simulink model "flightController"  (R2022a)
settings: Solver=ode3  StartTime=0  StopTime=TFinal  FixedStep=Ts  RelTol=1e-3  EnableMultiTasking=on
undefined symbols (not defined in the file): Controller, DiscIntNeverNeededParam, Ts, Vehicle
libraries: vrlib x2, dspfdesign x1
(part 2 of 2)

== system flightController/Flight Controller1/LADRC - Roll ==
  y : Inport
  r : Inport  Port=2
  Demux : Demux  Outputs=3
  Digital Clock : DigitalClock  SampleTime=Ts
  Discrete-Time Integrator : DiscreteIntegrator  InitialCondition=[0 0 0]'  SampleTime=Ts  OutDataTypeStr=single  ICPrevOutput=DiscIntNeverNeededParam  ICPrevScaledInput=DiscIntNeverNeededParam
  Divide : Product  Inputs=*/  OutDataTypeStr=single
  Gain1 : Gain  Gain=2  OutDataTypeStr=single
  GreaterThan : RelationalOperator  Operator=>  OutDataTypeStr=boolean  RndMeth=Simplest  InputSameDT=off
  LESO : MATLAB Function  TreatAsAtomicUnit=on
  Product : Product  OutDataTypeStr=single
  Product1 : Product  OutDataTypeStr=single
  SaturationThrust : Saturate  UpperLimit=4*Controller.totalThrustMaxRelative*Controller.motorsThrustPerMotorMax  LowerLimit=-4*Controller.totalThrustMaxRelative*Controller.motorsThrustPerMotorMax  OutDataTypeStr=single
  Square : Math  Operator=square
  Sum1 : Sum  Inputs=+-|
  Sum2 : Sum  Inputs=|+-
  Sum3 : Sum  Inputs=+-|
  Switch : Switch  Criteria=u2 ~= 0  Threshold=0.1  SaturateOnIntegerOverflow=off  InputSameDT=off
  b : Constant  Value=10000  OutDataTypeStr=single
  t_warm : Constant  Value=0.1  OutDataTypeStr=single
  u_ini : Constant  Value=0  OutDataTypeStr=single
  wc : Constant  Value=12  OutDataTypeStr=single
  wo : Constant  Value=40  OutDataTypeStr=single
  u : Outport
  wires:
  LESO/1(z_dot) -> Discrete-Time Integrator/1
  Discrete-Time Integrator/1 -> LESO/1(z), Demux/1
  Demux/1 -> Sum3/2  "z1"
  Product/1 -> Sum1/1
  Sum1/1 -> Sum2/1  "u_0"
  Demux/3 -> Sum2/2  "z3"
  Sum2/1 -> Divide/1
  Square/1 -> Product/1
  Gain1/1 -> Product1/1
  Demux/2 -> Product1/2  "z2"
  Product1/1 -> Sum1/2
  SaturationThrust/1 -> LESO/5(u), u/1  "u"
  Switch/1 -> SaturationThrust/1
  Divide/1 -> Switch/1  "u"
  u_ini/1 -> Switch/3
  r/1 -> Sum3/1
  Sum3/1 -> Product/2
  b/1 -> LESO/3(b), Divide/2
  wc/1 -> Gain1/1, Square/1
  wo/1 -> LESO/2(wo)
  t_warm/1 -> GreaterThan/2
  Digital Clock/1 -> GreaterThan/1
  GreaterThan/1 -> Switch/2
  y/1 -> LESO/4(y)

== system flightController/Flight Controller1/LADRC - Yaw ==
  y : Inport
  r : Inport  Port=2
  Demux : Demux  Outputs=3
  Digital Clock : DigitalClock  SampleTime=Ts
  Discrete-Time Integrator : DiscreteIntegrator  InitialCondition=[0 0 0]'  SampleTime=Ts  OutDataTypeStr=single  ICPrevOutput=DiscIntNeverNeededParam  ICPrevScaledInput=DiscIntNeverNeededParam
  Divide : Product  Inputs=*/  OutDataTypeStr=single
  Gain1 : Gain  Gain=2  OutDataTypeStr=single
  GreaterThan : RelationalOperator  Operator=>  OutDataTypeStr=boolean  RndMeth=Simplest  InputSameDT=off
  LESO : MATLAB Function  TreatAsAtomicUnit=on
  Product : Product  OutDataTypeStr=single
  Product1 : Product  OutDataTypeStr=single
  SaturationThrust : Saturate  Commented=through  UpperLimit=0.001  LowerLimit=-0.001  OutDataTypeStr=single
  Scope : Scope  NumInputPorts=2
  Scope1 : Scope
  Square : Math  Operator=square
  Sum1 : Sum  Inputs=+-|
  Sum2 : Sum  Inputs=|+-
  Sum3 : Sum  Inputs=+-|
  Switch : Switch  Criteria=u2 ~= 0  Threshold=0.1  SaturateOnIntegerOverflow=off  InputSameDT=off
  b : Constant  Value=15000  OutDataTypeStr=single
  t_warm : Constant  Value=0.2  OutDataTypeStr=single
  u_ini : Constant  Value=0  OutDataTypeStr=single
  wc : Constant  Value=4  OutDataTypeStr=single
  wo : Constant  Value=14  OutDataTypeStr=single
  u : Outport
  wires:
  LESO/1(z_dot) -> Discrete-Time Integrator/1
  Discrete-Time Integrator/1 -> LESO/1(z), Demux/1
  Demux/1 -> Scope/1, Sum3/2  "z1"
  Product/1 -> Sum1/1
  Sum1/1 -> Sum2/1  "u_0"
  Demux/3 -> Sum2/2  "z3"
  Sum2/1 -> Divide/1
  Square/1 -> Product/1
  Gain1/1 -> Product1/1
  Demux/2 -> Product1/2  "z2"
  Product1/1 -> Sum1/2
  SaturationThrust/1 -> Scope1/1, LESO/5(u), u/1  "u"
  Switch/1 -> SaturationThrust/1
  Divide/1 -> Switch/1  "u"
  u_ini/1 -> Switch/3
  r/1 -> Sum3/1
  Sum3/1 -> Product/2
  b/1 -> Divide/2, LESO/3(b)
  wc/1 -> Gain1/1, Square/1
  wo/1 -> LESO/2(wo)
  t_warm/1 -> GreaterThan/2
  Digital Clock/1 -> GreaterThan/1
  GreaterThan/1 -> Switch/2
  y/1 -> Scope/2, LESO/4(y)

== system flightController/Flight Controller1/LADRC - dX ==
  y : Inport
  r : Inport  Port=2
  Constant : Constant  OutDataTypeStr=single
  Demux : Demux  Outputs=2
  Digital Clock : DigitalClock  SampleTime=Ts
  Discrete-Time Integrator : DiscreteIntegrator  InitialCondition=[0 0]'  SampleTime=Ts  ICPrevOutput=DiscIntNeverNeededParam  ICPrevScaledInput=DiscIntNeverNeededParam
  Divide : Product  Inputs=*/
  GreaterThan : RelationalOperator  Operator=>  OutDataTypeStr=boolean  RndMeth=Simplest  InputSameDT=off
  LESO - 1st order : MATLAB Function  TreatAsAtomicUnit=on
  Product : Product
  Saturation : Saturate  UpperLimit=pi/8  LowerLimit=-pi/8
  Sum1 : Sum  Inputs=+-|
  Sum3 : Sum  Inputs=+-|
  Switch : Switch  Criteria=u2 ~= 0  Threshold=0.1  SaturateOnIntegerOverflow=off  InputSameDT=off
  b : Gain  Gain=-20
  b1 : Gain  Gain=-30
  bw_c : Gain
  bw_c1 : Gain  Gain=2
  bw_o : Gain  Gain=3
  bw_o1 : Gain  Gain=6
  t_warm : Constant  Value=0.01
  u_ini : Constant  Value=0  OutDataTypeStr=single
  u : Outport
  wires:
  LESO - 1st order/1(z_dot) -> Discrete-Time Integrator/1
  Discrete-Time Integrator/1 -> LESO - 1st order/1(z), Demux/1
  Demux/1 -> Sum3/2  "z1"
  Product/1 -> Sum1/1
  Sum1/1 -> Divide/1  "u_0"
  Demux/2 -> Sum1/2  "z2"
  Saturation/1 -> u/1, LESO - 1st order/5(u)  "u"
  Divide/1 -> Switch/1  "u"
  u_ini/1 -> Switch/3
  r/1 -> Sum3/1
  Sum3/1 -> Product/2
  b/1 -> LESO - 1st order/3(b), Divide/2
  bw_c/1 -> Product/1
  bw_o/1 -> LESO - 1st order/2(wo)
  t_warm/1 -> GreaterThan/2
  Digital Clock/1 -> GreaterThan/1
  GreaterThan/1 -> Switch/2
  y/1 -> LESO - 1st order/4(y)
  Constant/1 -> bw_o/1, bw_c/1, b/1
  Switch/1 -> Saturation/1  "u"

== system flightController/Flight Controller1/LADRC - dY ==
  y : Inport
  r : Inport  Port=2
  Constant : Constant  OutDataTypeStr=single
  Demux : Demux  Outputs=2
  Digital Clock : DigitalClock  SampleTime=Ts
  Discrete-Time Integrator : DiscreteIntegrator  InitialCondition=[0 0]'  SampleTime=Ts  ICPrevOutput=DiscIntNeverNeededParam  ICPrevScaledInput=DiscIntNeverNeededParam
  Divide : Product  Inputs=*/
  GreaterThan : RelationalOperator  Operator=>  OutDataTypeStr=boolean  RndMeth=Simplest  InputSameDT=off
  LESO - 1st order : MATLAB Function  TreatAsAtomicUnit=on
  Product : Product
  Saturation : Saturate  UpperLimit=pi/8  LowerLimit=-pi/8
  Sum1 : Sum  Inputs=+-|
  Sum3 : Sum  Inputs=+-|
  Switch : Switch  Criteria=u2 ~= 0  Threshold=0.1  SaturateOnIntegerOverflow=off  InputSameDT=off
  b : Gain  Gain=20
  bw_c : Gain
  bw_o : Gain  Gain=3
  t_warm : Constant  Value=0.01
  u_ini : Constant  Value=0  OutDataTypeStr=single
  u : Outport
  wires:
  LESO - 1st order/1(z_dot) -> Discrete-Time Integrator/1
  Discrete-Time Integrator/1 -> LESO - 1st order/1(z), Demux/1
  Demux/1 -> Sum3/2  "z1"
  Product/1 -> Sum1/1
  Sum1/1 -> Divide/1  "u_0"
  Demux/2 -> Sum1/2  "z2"
  Saturation/1 -> u/1, LESO - 1st order/5(u)  "u"
  Divide/1 -> Switch/1  "u"
  u_ini/1 -> Switch/3
  r/1 -> Sum3/1
  Sum3/1 -> Product/2
  b/1 -> LESO - 1st order/3(b), Divide/2
  bw_c/1 -> Product/1
  bw_o/1 -> LESO - 1st order/2(wo)
  t_warm/1 -> GreaterThan/2
  Digital Clock/1 -> GreaterThan/1
  GreaterThan/1 -> Switch/2
  y/1 -> LESO - 1st order/4(y)
  Constant/1 -> bw_o/1, bw_c/1, b/1
  Switch/1 -> Saturation/1  "u"

== system flightController/Flight Controller1/LADRC - dZ ==
  y : Inport
  r : Inport  Port=2
  Demux : Demux  Outputs=3
  Digital Clock : DigitalClock  SampleTime=Ts
  Discrete LESO 2nd Order : MATLAB Function  TreatAsAtomicUnit=on
  Divide : Product  Inputs=*/  OutDataTypeStr=single
  Gain : Gain  Gain=3  OutDataTypeStr=single
  Gain1 : Gain  Gain=2  OutDataTypeStr=single
  GreaterThan : RelationalOperator  Operator=>  OutDataTypeStr=boolean  RndMeth=Simplest  InputSameDT=off
  Magnitude Limit : Saturate  UpperLimit=4*Controller.totalThrustMaxRelative*Controller.motorsThrustPerMotorMax  LowerLimit=-4*Controller.totalThrustMaxRelative*Controller.motorsThrustPerMotorMax  OutDataTypeStr=single
  Memory : Memory  InitialCondition=[0 0 380]'
  Memory1 : Memory  InitialCondition=-0.6
  Product : Product  OutDataTypeStr=single
  Product1 : Product  OutDataTypeStr=single
  Rate Limit : Saturate  UpperLimit=0.05  LowerLimit=-0.05
  Square : Math  Operator=square
  Sum : Sum  Inputs=|++
  Sum1 : Sum  Inputs=+-|
  Sum2 : Sum  Inputs=|+-
  Sum3 : Sum  Inputs=+-|
  Sum4 : Sum  Inputs=|+-
  Switch : Switch  Criteria=u2 ~= 0  Threshold=0.1  SaturateOnIntegerOverflow=off  InputSameDT=off
  b : Constant  Value=800  OutDataTypeStr=single
  t_warm : Constant  Value=0  OutDataTypeStr=single
  u_ini : Constant  Value=-1  OutDataTypeStr=single
  wc : Constant  Value=20  OutDataTypeStr=single
  u : Outport
  wires:
  Discrete LESO 2nd Order/1(z_out) -> Memory/1, Demux/1
  Demux/1 -> Sum3/2  "z1"
  Product/1 -> Sum1/1
  Sum1/1 -> Sum2/1  "u_0"
  Demux/3 -> Sum2/2  "z3"
  Sum2/1 -> Divide/1
  Square/1 -> Product/1
  Gain1/1 -> Product1/1
  Demux/2 -> Product1/2  "z2"
  Product1/1 -> Sum1/2
  Divide/1 -> Switch/1  "u"
  u_ini/1 -> Switch/3
  r/1 -> Sum3/1
  Sum3/1 -> Product/2
  b/1 -> Divide/2, Discrete LESO 2nd Order/2(b)
  wc/1 -> Gain/1, Square/1, Gain1/1
  Gain/1 -> Discrete LESO 2nd Order/3(wo)
  t_warm/1 -> GreaterThan/2
  Digital Clock/1 -> GreaterThan/1
  GreaterThan/1 -> Switch/2
  y/1 -> Discrete LESO 2nd Order/4(y)
  Memory/1 -> Discrete LESO 2nd Order/1(z_in)
  Memory1/1 -> Sum4/2, Discrete LESO 2nd Order/5(u), Sum/2
  Rate Limit/1 -> Sum/1
  Sum/1 -> Magnitude Limit/1
  Sum4/1 -> Rate Limit/1
  Switch/1 -> Sum4/1
  Magnitude Limit/1 -> u/1, Memory1/1

== system flightController/Flight Controller1/LADRC - dZ1 ==
  y : Inport
  r : Inport  Port=2
  Demux : Demux  Outputs=3
  Digital Clock : DigitalClock  SampleTime=Ts
  Discrete LESO 2nd Order : MATLAB Function  TreatAsAtomicUnit=on
  Divide : Product  Inputs=*/  OutDataTypeStr=single
  Gain : Gain  Gain=3  OutDataTypeStr=single
  Gain1 : Gain  Gain=2  OutDataTypeStr=single
  GreaterThan : RelationalOperator  Operator=>  OutDataTypeStr=boolean  RndMeth=Simplest  InputSameDT=off
  Magnitude Limit : Saturate  UpperLimit=4*Controller.totalThrustMaxRelative*Controller.motorsThrustPerMotorMax  LowerLimit=-4*Controller.totalThrustMaxRelative*Controller.motorsThrustPerMotorMax  OutDataTypeStr=single
  Memory : Memory  InitialCondition=[0 0 0]'
  Memory1 : Memory
  Product : Product  OutDataTypeStr=single
  Product1 : Product  OutDataTypeStr=single
  Rate Limit : Saturate  UpperLimit=0.05  LowerLimit=-0.05
  Square : Math  Operator=square
  Sum : Sum  Inputs=|++
  Sum1 : Sum  Inputs=+-|
  Sum2 : Sum  Inputs=|+-
  Sum3 : Sum  Inputs=+-|
  Sum4 : Sum  Inputs=|+-
  Switch : Switch  Criteria=u2 ~= 0  Threshold=0.1  SaturateOnIntegerOverflow=off  InputSameDT=off
  b : Constant  Value=10000  OutDataTypeStr=single
  t_warm : Constant  Value=0  OutDataTypeStr=single
  u_ini : Constant  Value=-1  OutDataTypeStr=single
  wc : Constant  Value=10  OutDataTypeStr=single
  u : Outport
  wires:
  Discrete LESO 2nd Order/1(z_out) -> Memory/1, Demux/1
  Demux/1 -> Sum3/2  "z1"
  Product/1 -> Sum1/1
  Sum1/1 -> Sum2/1  "u_0"
  Demux/3 -> Sum2/2  "z3"
  Sum2/1 -> Divide/1
  Square/1 -> Product/1
  Gain1/1 -> Product1/1
  Demux/2 -> Product1/2  "z2"
  Product1/1 -> Sum1/2
  Divide/1 -> Switch/1  "u"
  u_ini/1 -> Switch/3
  r/1 -> Sum3/1
  Sum3/1 -> Product/2
  b/1 -> Divide/2, Discrete LESO 2nd Order/2(b)
  wc/1 -> Gain/1, Square/1, Gain1/1
  Gain/1 -> Discrete LESO 2nd Order/3(wo)
  t_warm/1 -> GreaterThan/2
  Digital Clock/1 -> GreaterThan/1
  GreaterThan/1 -> Switch/2
  y/1 -> Discrete LESO 2nd Order/4(y)
  Memory/1 -> Discrete LESO 2nd Order/1(z_in)
  Memory1/1 -> Sum4/2, Discrete LESO 2nd Order/5(u), Sum/2
  Rate Limit/1 -> Sum/1
  Sum/1 -> Magnitude Limit/1
  Sum4/1 -> Rate Limit/1
  Switch/1 -> Sum4/1
  Magnitude Limit/1 -> u/1, Memory1/1

== system flightController/Flight Controller1/XBOX CONTROLLER ==
  Bus Creator : BusCreator  Inputs=8
  Bus Creator1 : BusCreator  Inputs=11
  Constant : Constant  Value=[0 0 0 0 0 0 0 0]
  Dead Zone{,1..3} (4 alike) : DeadZone  LowerValue=-0.18  UpperValue=0.18
  Demux : Demux  Outputs=8
  Demux1 : Demux  Outputs=11
  Gain : Gain  Gain=-1
  Gain1 : Gain
  Joystick Input : vrlib/Joystick Input  joyid=1  adjustports=on  forcefeed=off
  Analog : Outport
  Buttons : Outport  Port=2
  wires:
  Demux1/4 -> Bus Creator1/4  "Y"
  Dead Zone/1 -> Bus Creator/1  "LStick-X"
  Demux1/9 -> Bus Creator1/9  "XBOX"
  Demux1/1 -> Bus Creator1/1  "A"
  Demux1/10 -> Bus Creator1/10  "LStick"
  Demux1/5 -> Bus Creator1/5  "LB"
  Demux/7 -> Bus Creator/7  "DPad-X"
  Joystick Input/2 -> Demux1/1
  Demux/5 -> Dead Zone3/1  "RStick-Y"
  Demux/4 -> Dead Zone2/1  "RStick-X"
  Dead Zone2/1 -> Bus Creator/4  "RStick-X"
  Demux/3 -> Bus Creator/3  "LT"
  Demux/8 -> Bus Creator/8  "DPad-Y"
  Joystick Input/1 -> Demux/1
  Demux/6 -> Bus Creator/6  "RT"
  Dead Zone1/1 -> Gain1/1  "LStick-Y"
  Demux/1 -> Dead Zone/1  "LStick-X"
  Bus Creator1/1 -> Buttons/1  "Buttons"
  Gain/1 -> Bus Creator/5  "RStick-Y"
  Demux/2 -> Dead Zone1/1  "LStick-Y"
  Bus Creator/1 -> Analog/1  "Analog"
  Demux1/3 -> Bus Creator1/3  "X"
  Demux1/6 -> Bus Creator1/6  "RB"
  Demux1/7 -> Bus Creator1/7  "Back"
  Demux1/11 -> Bus Creator1/11  "RStick"
  Demux1/2 -> Bus Creator1/2  "B"
  Demux1/8 -> Bus Creator1/8  "Start"
  Dead Zone3/1 -> Gain/1  "RStick-Y"
  Gain1/1 -> Bus Creator/2  "LStick-Y"

== system flightController/Flight Controller1/thrustsToMotorCommands ==
  thrusts_refin : Inport
  1 : Constant  OutDataTypeStr=single
  10 : Constant  Value=10  OutDataTypeStr=single
  2 : Constant  Value=-1  OutDataTypeStr=single
  Digital Clock : DigitalClock  SampleTime=Ts
  Digital Clock1 : DigitalClock  SampleTime=Ts
  Gain : Gain  Gain=1/40  OutDataTypeStr=single
  GreaterThan : RelationalOperator  Operator=>  OutDataTypeStr=boolean  RndMeth=Simplest  InputSameDT=off
  MotorDirections : Gain  Gain=[1 -1 1 -1]
  Mux : Mux
  Product : Product  OutDataTypeStr=single
  Saturation : Saturate  UpperLimit=40  LowerLimit=0  OutDataTypeStr=single
  Saturation5 : Saturate  UpperLimit=Vehicle.Motor.maxLimit  LowerLimit=Vehicle.Motor.minLimit
  Scope : Scope
  Sum : Sum  Inputs=|+-
  Sum1 : Sum  Inputs=|-+
  Switch : Switch  Criteria=u2 ~= 0  Threshold=0.1  SaturateOnIntegerOverflow=off  InputSameDT=off
  ThrustToMotorCommand : Gain  Gain=-Vehicle.Motor.thrustToMotorCommand
  t_warm : Constant  Value=10  OutDataTypeStr=single
  motors_cmdout : Outport  VectorParamsAs1DForOutWhenUnconnected=off
  wires:
  Saturation5/1 -> Product/2, MotorDirections/1
  MotorDirections/1 -> Switch/3
  ThrustToMotorCommand/1 -> Saturation5/1
  thrusts_refin/1 -> ThrustToMotorCommand/1
  Product/1 -> Switch/1
  Switch/1 -> motors_cmdout/1
  GreaterThan/1 -> Switch/2
  Digital Clock/1 -> GreaterThan/1
  t_warm/1 -> GreaterThan/2
  Digital Clock1/1 -> Sum/1
  10/1 -> Sum/2
  Sum/1 -> Saturation/1
  Saturation/1 -> Gain/1
  1/1 -> Mux/3, Sum1/2
  2/1 -> Mux/2, Mux/4
  Sum1/1 -> Scope/1, Mux/1
  Mux/1 -> Product/1

== matlab function flightController/Flight Controller1/LADRC - Roll/LESO ==
  data: z input single size=[3 1]; wo input single; b input single; z_dot output single size=[3 1]; y input single; u input single
function z_dot = LESO(z, wo, b, y, u)
    A = [0 1 0; 0 0 1; 0 0 0];
    B = [0 b 0]';
    C = [1 0 0];
    L = [3*wo 3*wo^2 wo^3]';
        
    z_dot = A*z + B*u + L*(y-z(1));

== matlab function flightController/Flight Controller1/LADRC - Yaw/LESO ==
  data: z input single size=[3 1]; wo input single; b input single; z_dot output single size=[3 1]; y input single; u input single
function z_dot = LESO(z, wo, b, y, u)
    A = [0 1 0; 0 0 1; 0 0 0];
    B = [0 b 0]';
    C = [1 0 0];
    L = [3*wo 3*wo^2 wo^3]';
        
    z_dot = A*z + B*u + L*(y-z(1));

== matlab function flightController/Flight Controller1/LADRC - dX/LESO - 1st order ==
  data: z input single; wo input single; b input single; z_dot output single; y input single; u input single
function z_dot = LESO(z, wo, b, y, u)

% %     A = [zeros(2,1), eye(2); zeros(1,2+1)];
%     A = [0 1 0; 0 0 1; 0 0 0];
% %     B = [zeros(2-1, 1); b; 0];
%     B = [0 1 0]';
% %     L = poly(-wo * ones(1, 2+1));
% %     L = flip(L(2:end));
%     L = []
%     C = [1 0 0];

    A = [0 1; 0 0];
    B = [b 0]';
    L = [2*wo wo^2]';
        
    z_dot = A*z+ B*u + L*(y-z(1));

== matlab function flightController/Flight Controller1/LADRC - dY/LESO - 1st order ==
  data: z input single; wo input single; b input single; z_dot output single; y input single; u input single
function z_dot = LESO(z, wo, b, y, u)

% %     A = [zeros(2,1), eye(2); zeros(1,2+1)];
%     A = [0 1 0; 0 0 1; 0 0 0];
% %     B = [zeros(2-1, 1); b; 0];
%     B = [0 1 0]';
% %     L = poly(-wo * ones(1, 2+1));
% %     L = flip(L(2:end));
%     L = []
%     C = [1 0 0];

    A = [0 1; 0 0];
    B = [b 0]';
    L = [2*wo wo^2]';
        
    z_dot = A*z+ B*u + L*(y-z(1));

== matlab function flightController/Flight Controller/LADRC - dZ/Discrete LESO 2nd Order ==
  data: z_in input; b input single; wo input single; z_out output single size=[3 1]; y input single; u input single; Ts parameter
function z_out = DLESO(z_in, b, wo, y, u, Ts)
%     
%     persistent count
%     if isempty(count)
%         count = single(0);
%     end

    A = [1 Ts Ts^2/2; 0 1 Ts; 0 0 1];
    B = [b*Ts^2/2 b*Ts 0]';
    C = [1 0 0];
    z_eso = exp(-wo*Ts);
    L = [1-(z_eso)^3 (3/(2*Ts))*(1-z_eso)^2*(1+z_eso) (1/Ts^2)*(1-z_eso)^3]';
    
%     if count == 0
%         z_out = (A - L*C*A)*z_init + (B - L*C*B)*-1 + L*y;
%         count = single(1);
%     else
    z_out = (A - L*C*A)*z_in + (B - L*C*B)*u + L*y;
%     end

== matlab function flightController/Flight Controller1/LADRC - dZ/Discrete LESO 2nd Order ==
  data: z_in input; b input single; wo input single; z_out output single size=[3 1]; y input single; u input single; Ts parameter
function z_out = DLESO(z_in, b, wo, y, u, Ts)
%     
%     persistent count
%     if isempty(count)
%         count = single(0);
%     end

    A = [1 Ts Ts^2/2; 0 1 Ts; 0 0 1];
    B = [b*Ts^2/2 b*Ts 0]';
    C = [1 0 0];
    z_eso = exp(-wo*Ts);
    L = [1-(z_eso)^3 (3/(2*Ts))*(1-z_eso)^2*(1+z_eso) (1/Ts^2)*(1-z_eso)^3]';
    
%     if count == 0
%         z_out = (A - L*C*A)*z_init + (B - L*C*B)*-1 + L*y;
%         count = single(1);
%     else
    z_out = (A - L*C*A)*z_in + (B - L*C*B)*u + L*y;
%     end

== matlab function flightController/Flight Controller1/LADRC - dZ1/Discrete LESO 2nd Order ==
  data: z_in input; b input single; wo input single; z_out output single size=[3 1]; y input single; u input single; Ts parameter
function z_out = DLESO(z_in, b, wo, y, u, Ts)
%     
%     persistent count
%     if isempty(count)
%         count = single(0);
%     end

    A = [1 Ts Ts^2/2; 0 1 Ts; 0 0 1];
    B = [b*Ts^2/2 b*Ts 0]';
    C = [1 0 0];
    z_eso = exp(-wo*Ts);
    L = [1-(z_eso)^3 (3/(2*Ts))*(1-z_eso)^2*(1+z_eso) (1/Ts^2)*(1-z_eso)^3]';
    
%     if count == 0
%         z_out = (A - L*C*A)*z_init + (B - L*C*B)*-1 + L*y;
%         count = single(1);
%     else
    z_out = (A - L*C*A)*z_in + (B - L*C*B)*u + L*y;
%     end

== matlab function flightController/Flight Controller/LADRC - dX/Discrete LESO 1st Order ==
  data: z_in input; b input single; wo input single; z_out output single size=[2 1]; y input single; u input single; Ts parameter
function z_out = DLESO(z_in, b, wo, y, u, Ts)


    A = [1 Ts; 0 1];
    B = [b*Ts 0]';
    C = [1 0];
    z_eso = exp(-wo*Ts);
    L = [1-(z_eso)^2 (1/Ts)*((1-z_eso)^2)]';
    
    z_out = (A - L*C*A)*z_in + (B - L*C*B)*u + L*y;

== matlab function flightController/Flight Controller - XBOX/LADRC - Roll/Discrete LESO 2nd Order ==
  data: z_in input; b input single; wo input single; z_out output single size=[3 1]; y input single; u input single; Ts parameter
function z_out = DLESO(z_in, b, wo, y, u, Ts)
%     
%     persistent count
%     if isempty(count)
%         count = single(0);
%     end

    A = [1 Ts Ts^2/2; 0 1 Ts; 0 0 1];
    B = [b*Ts^2/2 b*Ts 0]';
    C = [1 0 0];
    z_eso = exp(-wo*Ts);
    L = [1-(z_eso)^3 (3/(2*Ts))*(1-z_eso)^2*(1+z_eso) (1/Ts^2)*(1-z_eso)^3]';
    
%     if count == 0
%         z_out = (A - L*C*A)*z_init + (B - L*C*B)*-1 + L*y;
%         count = single(1);
%     else
    z_out = (A - L*C*A)*z_in + (B - L*C*B)*u + L*y;
%     end

== matlab function flightController/Flight Controller - XBOX/LADRC - Yaw/Discrete LESO 2nd Order ==
  data: z_in input; b input single; wo input single; z_out output single size=[3 1]; y input single; u input single; Ts parameter
function z_out = DLESO(z_in, b, wo, y, u, Ts)
%     
%     persistent count
%     if isempty(count)
%         count = single(0);
%     end

    A = [1 Ts Ts^2/2; 0 1 Ts; 0 0 1];
    B = [b*Ts^2/2 b*Ts 0]';
    C = [1 0 0];
    z_eso = exp(-wo*Ts);
    L = [1-(z_eso)^3 (3/(2*Ts))*(1-z_eso)^2*(1+z_eso) (1/Ts^2)*(1-z_eso)^3]';
    
%     if count == 0
%         z_out = (A - L*C*A)*z_init + (B - L*C*B)*-1 + L*y;
%         count = single(1);
%     else
    z_out = (A - L*C*A)*z_in + (B - L*C*B)*u + L*y;
%     end

== matlab function flightController/Flight Controller - XBOX/LADRC - dX/Discrete LESO 1st Order ==
  data: z_in input; b input single; wo input single; z_out output single size=[2 1]; y input single; u input single; Ts parameter
function z_out = DLESO(z_in, b, wo, y, u, Ts)


    A = [1 Ts; 0 1];
    B = [b*Ts 0]';
    C = [1 0];
    z_eso = exp(-wo*Ts);
    L = [1-(z_eso)^2 (1/Ts)*((1-z_eso)^2)]';
    
    z_out = (A - L*C*A)*z_in + (B - L*C*B)*u + L*y;

== matlab function flightController/Flight Controller - XBOX/LADRC - dY/Discrete LESO 1st Order ==
  data: z_in input; b input single; wo input single; z_out output single size=[2 1]; y input single; u input single; Ts parameter
function z_out = DLESO(z_in, b, wo, y, u, Ts)


    A = [1 Ts; 0 1];
    B = [b*Ts 0]';
    C = [1 0];
    z_eso = exp(-wo*Ts);
    L = [1-(z_eso)^2 (1/Ts)*((1-z_eso)^2)]';
    
    z_out = (A - L*C*A)*z_in + (B - L*C*B)*u + L*y;

== matlab function flightController/Flight Controller - XBOX/LADRC - dZ/Discrete LESO 2nd Order ==
  data: z_in input; b input single; wo input single; z_out output single size=[3 1]; y input single; u input single; Ts parameter
function z_out = DLESO(z_in, b, wo, y, u, Ts)
%     
%     persistent count
%     if isempty(count)
%         count = single(0);
%     end

    A = [1 Ts Ts^2/2; 0 1 Ts; 0 0 1];
    B = [b*Ts^2/2 b*Ts 0]';
    C = [1 0 0];
    z_eso = exp(-wo*Ts);
    L = [1-(z_eso)^3 (3/(2*Ts))*(1-z_eso)^2*(1+z_eso) (1/Ts^2)*(1-z_eso)^3]';
    
%     if count == 0
%         z_out = (A - L*C*A)*z_init + (B - L*C*B)*-1 + L*y;
%         count = single(1);
%     else
    z_out = (A - L*C*A)*z_in + (B - L*C*B)*u + L*y;
%     end

== matlab function flightController/Flight Controller/LADRC - Pitch/Discrete LESO 2nd Order ==
  data: z_in input; b input single; wo input single; z_out output single size=[3 1]; y input single; u input single; Ts parameter
function z_out = DLESO(z_in, b, wo, y, u, Ts)
%     
%     persistent count
%     if isempty(count)
%         count = single(0);
%     end

    A = [1 Ts Ts^2/2; 0 1 Ts; 0 0 1];
    B = [b*Ts^2/2 b*Ts 0]';
    C = [1 0 0];
    z_eso = exp(-wo*Ts);
    L = [1-(z_eso)^3 (3/(2*Ts))*(1-z_eso)^2*(1+z_eso) (1/Ts^2)*(1-z_eso)^3]';
    
%     if count == 0
%         z_out = (A - L*C*A)*z_init + (B - L*C*B)*-1 + L*y;
%         count = single(1);
%     else
    z_out = (A - L*C*A)*z_in + (B - L*C*B)*u + L*y;
%     end

== matlab function flightController/Flight Controller/LADRC - dX1/Discrete LESO 1st Order ==
  data: z_in input; b input single; wo input single; z_out output single size=[2 1]; y input single; u input single; Ts parameter
function z_out = DLESO(z_in, b, wo, y, u, Ts)


    A = [1 Ts; 0 1];
    B = [b*Ts 0]';
    C = [1 0];
    z_eso = exp(-wo*Ts);
    L = [1-(z_eso)^2 (1/Ts)*((1-z_eso)^2)]';
    
    z_out = (A - L*C*A)*z_in + (B - L*C*B)*u + L*y;

== matlab function flightController/Flight Controller/LADRC - dX/MATLAB Function ==
  data: v_1 input; out output; v_2 input; r_0 input; h_0 input
function out = fhan(v_1, v_2, r_0, h_0)

d = h_0 * r_0^2;
a_0 = h_0 * v_2;
y = v_1 + a_0;
a_1 = sqrt(d*(d + 8*norm(y)));
a_2 = a_0 + sign(y)*(a_1 - d)/2;
s_y = (sign(y + d) - sign(y-d))/2;
a = (a_0 + y - a_2)*s_y + a_2;
s_a = (sign(a+d) - sign(a-d))/2;

out = -r_0*(a/d - sign(a))*s_a - r_0*sign(0);

== matlab function flightController/Flight Controller - XBOX/LADRC - Pitch/Discrete LESO 2nd Order ==
  data: z_in input; b input single; wo input single; z_out output single size=[3 1]; y input single; u input single; Ts parameter
function z_out = DLESO(z_in, b, wo, y, u, Ts)
%     
%     persistent count
%     if isempty(count)
%         count = single(0);
%     end

    A = [1 Ts Ts^2/2; 0 1 Ts; 0 0 1];
    B = [b*Ts^2/2 b*Ts 0]';
    C = [1 0 0];
    z_eso = exp(-wo*Ts);
    L = [1-(z_eso)^3 (3/(2*Ts))*(1-z_eso)^2*(1+z_eso) (1/Ts^2)*(1-z_eso)^3]';
    
%     if count == 0
%         z_out = (A - L*C*A)*z_init + (B - L*C*B)*-1 + L*y;
%         count = single(1);
%     else
    z_out = (A - L*C*A)*z_in + (B - L*C*B)*u + L*y;
%     end

== matlab function flightController/Flight Controller/LADRC - Roll/Discrete LESO 2nd Order ==
  data: z_in input; b input single; wo input single; z_out output single size=[3 1]; y input single; u input single; Ts parameter
function z_out = DLESO(z_in, b, wo, y, u, Ts)
%     
%     persistent count
%     if isempty(count)
%         count = single(0);
%     end

    A = [1 Ts Ts^2/2; 0 1 Ts; 0 0 1];
    B = [b*Ts^2/2 b*Ts 0]';
    C = [1 0 0];
    z_eso = exp(-wo*Ts);
    L = [1-(z_eso)^3 (3/(2*Ts))*(1-z_eso)^2*(1+z_eso) (1/Ts^2)*(1-z_eso)^3]';
    
%     if count == 0
%         z_out = (A - L*C*A)*z_init + (B - L*C*B)*-1 + L*y;
%         count = single(1);
%     else
    z_out = (A - L*C*A)*z_in + (B - L*C*B)*u + L*y;
%     end

== matlab function flightController/Flight Controller/LADRC - Yaw/Discrete LESO 2nd Order ==
  data: z_in input; b input single; wo input single; z_out output single size=[3 1]; y input single; u input single; Ts parameter
function z_out = DLESO(z_in, b, wo, y, u, Ts)
%     
%     persistent count
%     if isempty(count)
%         count = single(0);
%     end

    A = [1 Ts Ts^2/2; 0 1 Ts; 0 0 1];
    B = [b*Ts^2/2 b*Ts 0]';
    C = [1 0 0];
    z_eso = exp(-wo*Ts);
    L = [1-(z_eso)^3 (3/(2*Ts))*(1-z_eso)^2*(1+z_eso) (1/Ts^2)*(1-z_eso)^3]';
    
%     if count == 0
%         z_out = (A - L*C*A)*z_init + (B - L*C*B)*-1 + L*y;
%         count = single(1);
%     else
    z_out = (A - L*C*A)*z_in + (B - L*C*B)*u + L*y;
%     end

== matlab function flightController/Flight Controller1/LADRC - Pitch/LESO ==
  data: z input single size=[3 1]; wo input single; b input single; z_dot output single size=[3 1]; y input single; u input single
function z_dot = LESO(z, wo, b, y, u)
    A = [0 1 0; 0 0 1; 0 0 0];
    B = [0 b 0]';
    C = [1 0 0];
    L = [3*wo 3*wo^2 wo^3]';
        
    z_dot = A*z + B*u + L*(y-z(1));
